simulink model "Main_bikesim"  (R2023b)
settings: Solver=FixedStepAuto  StartTime=0.0  StopTime=sim_time-0.02  FixedStep=0.005
values from neighbouring files (symbols this model uses):
  A_d = (eye(size(A))+Ts*A)    [Main_sim.m]
  Ad_t = (eye(size(A_t))+Ts*A_t)    [Main_sim.m]
  B_d = Ts*B    [Main_sim.m]
  Bd_t = B_t*Ts    [Main_sim.m]
  bike_model = 1    [Main_sim.m]
  bike_params = LoadBikeParameters(bike)    [Main_sim.m]
  C1 = [1 0 0 0 0 0 0 ... (first row only)    [Main_sim.m]
  C2 = [(-g+((-h_imu*g)/h)) 0 (-h_imu*(h*v^2-(g*lr*c)))*sin(lambda)/((lr+lf)*h^2)+(v^2)*sin(lambda)/(lr+lf) 0 ... (first row only)    [Main_sim.m]
  counter = (Ts_GPS / Ts) - 1    (= 9)    [Main_sim.m]
  D1 = [0 0 (-h_imu*lr*v)/((lr+lf)*h) 0 0 0 0]'    [Main_sim.m]
  D2 = [(-h_imu*lr*v)/((lr+lf)*h) 0 0 0 0]'    [Main_sim.m]
  e1_max = abs(-k2*e2_max/k1)    [Main_sim.m]
  g = 9.81    [Main_sim.m]
  hor_dis = 10    [Main_sim.m]
  I_balancing_outer = 0.0    (= 0)    [Main_sim.m]
  initial_state_estimate = initial_state    [Main_sim.m]
  k1 = K(1)    [Main_sim.m]
  k2 = K(2)    [Main_sim.m]
  Kalman_gain1 = Kalman_gain1'    [Main_sim.m]
  Kalman_gain2 = Kalman_gain1(4:7,3:7)    [Main_sim.m]
  P_balancing_inner = 75.5    [Main_sim.m]
  P_balancing_outer = 75.75    [Main_sim.m]
  Psiref = traj(3:end,3)    [Main_sim.m]    (also in ReferenceGenerator.m = [Psiref(1); Psiref(1); Psiref])
  ref_dis = 0.01    [Main_sim.m]
  ref_start_idx = 2    [Main_sim.m]
  T = Rz*Ry*Rx    [Main_sim.m]
  Ts = 0.01    [Main_sim.m]
  v = 1.10    (= 1.1)    [Main_sim.m]
  Xref = traj(3:end,1)    [Main_sim.m]    (also in ReferenceGenerator.m = [Xref(1); Xref])
  Yref = traj(3:end,2)    [Main_sim.m]    (also in ReferenceGenerator.m = [Yref(1); Yref])
undefined symbols (not defined in the file or in its folder): C_t, D_t, initial_state, linearized_sys, pert_deltadot_state, pert_deltadot_state_fun, pert_phidot_state, pert_phidot_state_fun, sigbuilder_block
libraries: simulink x8, slpidlib x2, eeGeneralControl x1
(part 1 of 2)
settings Model: PauseTimes=0.16  Creator=Hadi Hajieghrary  LastModifiedBy=nicholasgranlund
settings SolverCC: MaxConsecutiveMinStep=10  ZeroCrossAlgorithm=Adaptive  AlgebraicLoopSolver=TrustRegion  AutoInsertRateTranBlk=on
settings OptimizationCC: ReuseModelBlockBuffer=off
settings DebuggingCC: AlgebraicLoopMsg=none  UnconnectedInputMsg=warning  UnconnectedOutputMsg=warning  UnconnectedLineMsg=warning
settings ModelReferenceCC: EnableRefExpFcnMdlSchedulingChecks=on
settings RTWCC: GenCodeOnly=on  DLArmComputeVersion=19.05

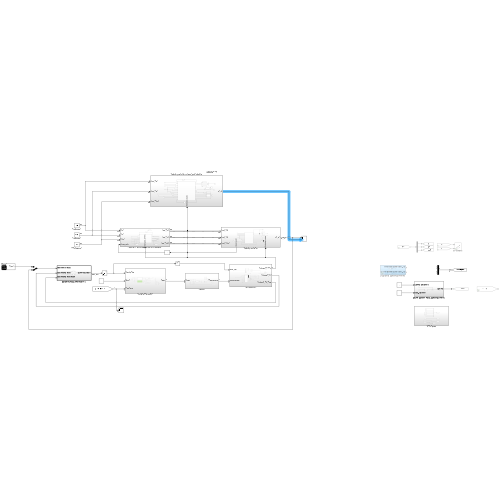
[thumbnail: Simulink's stored preview of the top-level diagram]
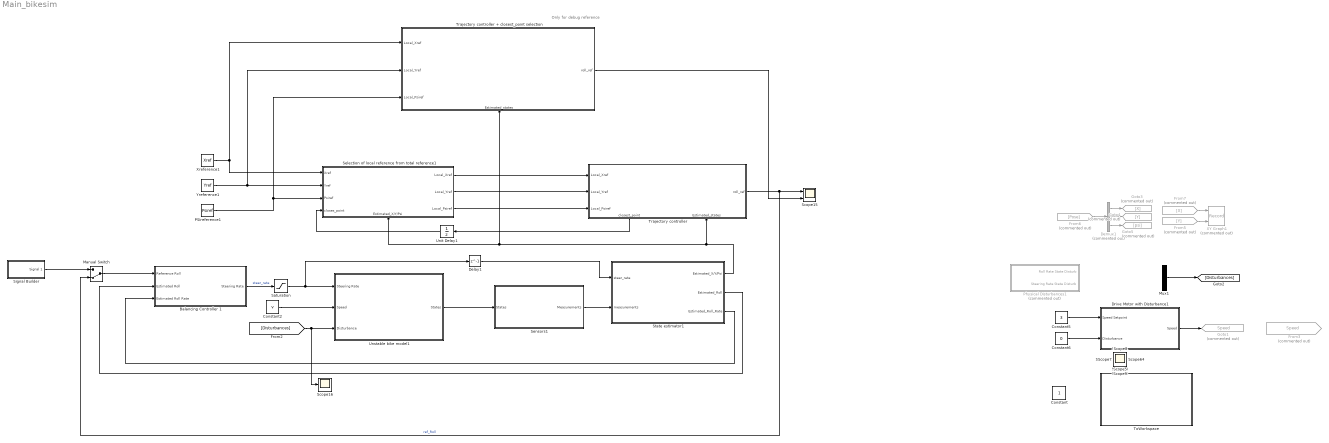
== system Main_bikesim ==
  note: Only for debug reference
  Balancing Controller 1 : Subsystem  TreatAsAtomicUnit=on  SystemSampleTime=Ts
      settings: MinAlgLoopOccurrences=on
  Constant2 : Constant  Value=v
  Constant5 : Constant  Value=3
  Constant6 : Constant  Value=0
  Delay1 : Delay  DelayLength=1  SampleTime=Ts
  Demux1 : Demux  Commented=on  Outputs=3
  Drive Motor with Disturbance1 : Subsystem
  From3 : From  Commented=on  GotoTag=Speed  TagVisibility=global
  From5 : From  Commented=on  GotoTag=Y
  From6 : From  Commented=on  GotoTag=Pose
  From7 : From  Commented=on  GotoTag=X
  Goto1 : Goto  Commented=on  GotoTag=Speed  TagVisibility=global
  Goto3 : Goto  Commented=on  GotoTag=X
  Goto4 : Goto  Commented=on  GotoTag=Y
  Goto5 : Goto  Commented=on  GotoTag=psi
  Manual Switch : ManualSwitch  CurrentSetting=0
  Mux1 : Mux  Inputs=2
  PSIreference1 : Constant  Value=Psiref
  Physical Disturbances1 : Subsystem  Commented=on
  Saturation : Saturate  UpperLimit=deg2rad(336/2)  LowerLimit=-deg2rad(336/2)
  Scope15 : Scope  NumInputPorts=2
  Scope{,1..14,16} (16 alike) : Scope
  Selection of local reference from total reference1 : Subsystem
      settings: PortSchema="{\"entries\":[{\"content\":{\"sides\":[{\"content\":{\"connectorIds\":[\"In1\",\"In2\",\"In3\",\"In4\"]},\"type\":\"ConnectorPlacement.EquallySpacedRectSide\",\"uuid\":\"b129a8ce-0ab0-4745-b919-7f1f6310ba72\"},{\"content\":{\"connectorIds\":[\"Out1\",\"Out2\",\"Out3\"],\"side\":\"RIGHT\"},\"type\":\"ConnectorPlacement.EquallySpacedRectSide\",\"uuid\":\"29e87fb1-7c56-4cac-b724-1406f2c9c629\"},{\"content\":{\"connectorIds\":[],\"side\":\"TOP\"},\"type\":\"ConnectorPlacement.EquallySpacedRectSide\",\"uuid\":\"7b58316d-0623-4272-bbb4-c0141a57ab8b\"},{\"content\":{\"connectorIds\":[\"In5\"],\"side\":\"BOTTOM\"},\"type\":\"ConnectorPlacement.EquallySpacedRectSide\",\"uuid\":\"0102ebd0-fd1a-417a-bd7a-ba724799aedf\"}]},\"type\":\"ConnectorPlacement.EquallySpacedConnector\",\"uuid\":\"fda0eb97-4558-45cb-9afe-cb94e226b238\"}],\"packageUris\":[\"http://schema.mathworks.com/mf0/Connector/R2020b\"],\"version\":\"1.0\"}"
  Sensors1 : Subsystem
  Signal Builder : Subsystem  Tag=STV Subsys  LoadFcn=sigbuilder_block('load');  StartFcn=sigbuilder_block('start');  StopFcn=sigbuilder_block('stop');  ClipboardFcn=sigbuilder_block('clipboard');  mask(Sigbuilder block){tuvar=[0:10]}
      mask help: Simulink:masks:SigbuilderBlock_MD
      mask init:
      | if ~strcmp(get_param(bdroot(gcbh),'SimulationStatus'),'stopped') tuvar = sigbuilder_block('maskInit'); end
      settings: CopyFcn=sigbuilder_block('copy');  DeleteFcn=sigbuilder_block('delete');  ModelCloseFcn=sigbuilder_block('modelClose');  PreSaveFcn=sigbuilder_block('preSave');  PauseFcn=sigbuilder_block('pause');  ContinueFcn=sigbuilder_block('continue');  NameChangeFcn=sigbuilder_block('namechange');  OpenFcn=sigbuilder_block('open',[418.8 162 550.8 400.2 ]);  CloseFcn=sigbuilder_block('close');
      mask Display: plot(0, 0, 100, 100,[2, 2, 32, 32, 2], [68, 8, 8, 68, 68],[32, 2], [38, 38], [32, 19, 2],[53, 60, 44], [32, 17, 17, 2],[16, 16, 31, 31]);txt = getActiveGroup(gcbh);text(2, 100, txt,'verticalAlignment', 'top');
  State estimator1 : Subsystem
  ToWorkspace : Subsystem
  Trajectory controller : Subsystem
      settings: PortSchema="{\"entries\":[{\"content\":{\"sides\":[{\"content\":{\"connectorIds\":[\"In1\",\"In2\",\"In3\"]},\"type\":\"ConnectorPlacement.EquallySpacedRectSide\",\"uuid\":\"e7a2fb02-f6cc-45e9-8980-79d12a8832e3\"},{\"content\":{\"connectorIds\":[\"Out1\"],\"side\":\"RIGHT\"},\"type\":\"ConnectorPlacement.EquallySpacedRectSide\",\"uuid\":\"304c1e91-f1f4-462f-993e-75a0bfc51b31\"},{\"content\":{\"connectorIds\":[],\"side\":\"TOP\"},\"type\":\"ConnectorPlacement.EquallySpacedRectSide\",\"uuid\":\"75b9e2ee-7eae-4db3-b507-7ba54d105139\"},{\"content\":{\"connectorIds\":[\"Out2\",\"In4\"],\"side\":\"BOTTOM\"},\"type\":\"ConnectorPlacement.EquallySpacedRectSide\",\"uuid\":\"8b853725-4c9a-4fb3-93ea-b9b3b3cf0d57\"}]},\"type\":\"ConnectorPlacement.EquallySpacedConnector\",\"uuid\":\"c24d7268-89b5-4c3c-b432-105407319c62\"}],\"packageUris\":[\"http://schema.mathworks.com/mf0/Connector/R2020b\"],\"version\":\"1.0\"}"
  Trajectory controller + closest_point selection : Subsystem
      settings: PortSchema="{\"entries\":[{\"content\":{\"sides\":[{\"content\":{\"connectorIds\":[\"In1\",\"In2\",\"In3\"]},\"type\":\"ConnectorPlacement.EquallySpacedRectSide\",\"uuid\":\"4e12ce37-1515-428d-8e72-ea3bf7cb0ff9\"},{\"content\":{\"connectorIds\":[\"Out1\"],\"side\":\"RIGHT\"},\"type\":\"ConnectorPlacement.EquallySpacedRectSide\",\"uuid\":\"a9718efd-1612-4f51-92cf-6f7a8bfe2bda\"},{\"content\":{\"connectorIds\":[],\"side\":\"TOP\"},\"type\":\"ConnectorPlacement.EquallySpacedRectSide\",\"uuid\":\"2b79877e-8290-4d72-b67b-1728e8961ce6\"},{\"content\":{\"connectorIds\":[\"In4\"],\"side\":\"BOTTOM\"},\"type\":\"ConnectorPlacement.EquallySpacedRectSide\",\"uuid\":\"2cd29579-a861-4f37-a88d-667717891393\"}]},\"type\":\"ConnectorPlacement.EquallySpacedConnector\",\"uuid\":\"1636a1cb-255f-43a6-9614-48f01e829aec\"}],\"packageUris\":[\"http://schema.mathworks.com/mf0/Connector/R2020b\"],\"version\":\"1.0\"}"
  Unit Delay1 : UnitDelay  InitialCondition=ref_start_idx  SampleTime=Ts  HasFrameUpgradeWarning=on
  Unstable bike model1 : Subsystem
  XY Graph1 : Record  Commented=on  FileSettingsInternal="{\"entries\":[{\"content\":{\"excelSettings\":{\"content\":{},\"type\":\"Streamout.ExcelSettings\"}},\"type\":\"Streamout.FileSettingStorage\",\"uuid\":\"\"}],\"packageUris\":[\"http:\\/\\/schema.mathworks.com\\/mf0\\/streamout_blocks\\/R2020a\"],\"version\":\"1.0\"}"  Layout=[1 1]  SignalsInternal="{\"entries\":[{\"content\":{},\"type\":\"RecordBlkView.InputSignals\",\"uuid\":\"\"}],\"packageUris\":[\"http:\\/\\/schema.mathworks.com\\/mf0\\/streamout_blocks\\/R2020a\"],\"version\":\"1.0\"}"  VisualizationBindings="{\"xyplotplugin\":{\"info\":[{\"series\":[],\"subplotID\":1}]}}"  CompatibilityTag=XY
  Xreference1 : Constant  Value=Xref
  Yreference1 : Constant  Value=Yref
  Constant : Constant  IOType=siggen
  wires:
  Yreference1/1 -> Trajectory controller + closest_point selection/2(Local_Yref), Selection of local reference from total reference1/2(Yref)
  State estimator1/1(Estimated_X/Y/Psi) -> Trajectory controller/4(Estimated_states), Selection of local reference from total reference1/5(Estimated_X/Y/Psi), Trajectory controller + closest_point selection/4(Estimated_states)
  PSIreference1/1 -> Trajectory controller + closest_point selection/3(Local_Psiref), Selection of local reference from total reference1/3(Psiref)
  Delay1/1 -> State estimator1/1(steer_rate)
  Unstable bike model1/1(States) -> Sensors1/1(States)
  Demux1/1 -> Goto3/1
  Balancing Controller 1/1(Steering Rate) -> Saturation/1  "steer_rate"
  Xreference1/1 -> Selection of local reference from total reference1/1(Xref), Trajectory controller + closest_point selection/1(Local_Xref)
  Selection of local reference from total reference1/3(Local_Psiref) -> Trajectory controller/3(Local_Psiref)
  Selection of local reference from total reference1/2(Local_Yref) -> Trajectory controller/2(Local_Yref)
  From5/1 -> XY Graph1/2
  Sensors1/1(Measurements) -> State estimator1/2(measurements)
  [Disturbances] -> Unstable bike model1/3(Disturbance), Scope16/1
  Trajectory controller/2(closest_point) -> Unit Delay1/1
  Selection of local reference from total reference1/1(Local_Xref) -> Trajectory controller/1(Local_Xref)
  State estimator1/2(Estimated_Roll) -> Balancing Controller 1/2(Estimated Roll)
  Demux1/3 -> Goto5/1
  Unit Delay1/1 -> Selection of local reference from total reference1/4(closes_point)
  Demux1/2 -> Goto4/1
  Drive Motor with Disturbance1/1(Speed) -> Goto1/1
  Mux1/1 -> [Disturbances]
  Constant5/1 -> Drive Motor with Disturbance1/1(Speed Setpoint)
  From7/1 -> XY Graph1/1
  Constant6/1 -> Drive Motor with Disturbance1/2(Disturbance)
  From6/1 -> Demux1/1
  State estimator1/3(Estimated_Roll_Rate) -> Balancing Controller 1/3(Estimated Roll Rate)
  Trajectory controller + closest_point selection/1(roll_ref) -> Scope15/2
  Manual Switch/1 -> Balancing Controller 1/1(Reference Roll)
  Signal Builder/1(Signal 1) -> Manual Switch/1
  Trajectory controller/1(roll_ref) -> Manual Switch/2, Scope15/1  "ref_Roll"
  Constant2/1 -> Unstable bike model1/2(Speed)
  Saturation/1 -> Delay1/1, Unstable bike model1/1(Steering Rate)

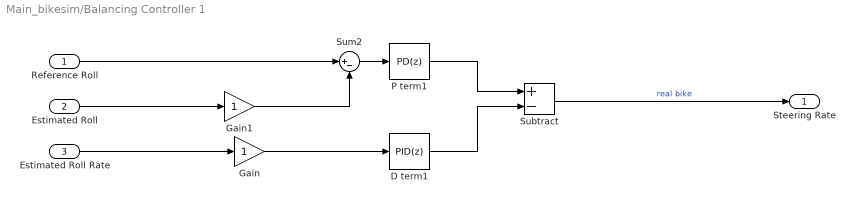
== system Main_bikesim/Balancing Controller 1 ==
  Reference Roll : Inport
  Estimated Roll : Inport  Port=2
  Estimated Roll Rate : Inport  Port=3
  D term1 : slpidlib/PID Controller  Controller=PID  Form=Parallel  TimeDomain=Discrete-time  UseExternalTs=off  SampleTime=Ts  IntegratorMethod=Forward Euler  FilterMethod=Forward Euler  ControllerParametersSource=internal  P=P_balancing_inner  I=0  UseKiTs=off  D=0  N=100  UseFilter=off  TunerSelectOption=Transfer Function Based (PID Tuner App)  InitialConditionSource=internal  InitialConditionForIntegrator=0  InitialConditionForFilter=0  DifferentiatorICPrevScaledInput=0  ExternalReset=none  TrackingMode=off  Kt=1  LimitOutput=off  SatLimitsSource=internal  UpperSaturationLimit=inf  LowerSaturationLimit=-inf  LinearizeAsGain=on  AntiWindupMode=none  Kb=1  LimitIntegrator=off  UpperIntegratorSaturationLimit=inf  LowerIntegratorSaturationLimit=-inf  POutMin=[]  POutMax=[]  IOutMin=[]  IOutMax=[]  DOutMin=[]  DOutMax=[]  NOutMin=[]  NOutMax=[]  SumOutMin=[]  SumOutMax=[]  SaturationOutMin=[]  SaturationOutMax=[]  PParamMin=[]  PParamMax=[]  IParamMin=[]  IParamMax=[]  DParamMin=[]  DParamMax=[]  NParamMin=[]  NParamMax=[]  KbParamMin=[]  KbParamMax=[]  KtParamMin=[]  KtParamMax=[]  KbOutMin=[]  KbOutMax=[]  KtOutMin=[]  KtOutMax=[]  IntegratorOutMin=[]  IntegratorOutMax=[]  FilterOutMin=[]  FilterOutMax=[]  SumI1OutMin=[]  SumI1OutMax=[]  SumI2OutMin=[]  SumI2OutMax=[]  SumI3OutMin=[]  SumI3OutMax=[]  SumI4OutMin=[]  SumI4OutMax=[]  SumDOutMin=[]  SumDOutMax=[]  DifferentiatorOutMin=[]  DifferentiatorOutMax=[]  FilterDiffOutCoefMin=[]  FilterDiffOutCoefMax=[]  ReciprocalOutMin=[]  ReciprocalOutMax=[]  SumDenOutMin=[]  SumDenOutMax=[]  SumNumOutMin=[]  SumNumOutMax=[]  DivideOutMin=[]  DivideOutMax=[]  UdiffTsProdOutMin=[]  UdiffTsProdOutMax=[]  NTsProdOutMin=[]  NTsProdOutMax=[]  UintegralTsProdOutMin=[]  UintegralTsProdOutMax=[]  UngainTsProdOutMin=[]  UngainTsProdOutMax=[]  ClampingZeroOutDataTypeStr=Inherit: Inherit via back propagation  ClampingZeroOutMin=[]  ClampingZeroOutMax=[]  FilterDenConstantOutDataTypeStr=Inherit: Inherit via back propagation  FilterDenConstantOutMin=[]  FilterDenConstantOutMax=[]  PCopyOutDataTypeStr=Inherit: Inherit via back propagation  PCopyOutMin=[]  PCopyOutMax=[]  NCopyOutDataTypeStr=Inherit: Inherit via back propagation  NCopyOutMin=[]  NCopyOutMax=[]  IntegratorContinuousStateAttributes=''  IntegratorStateMustResolveToSignalObject=off  IntegratorRTWStateStorageClass=Auto  FilterContinuousStateAttributes=''  FilterStateMustResolveToSignalObject=off  FilterRTWStateStorageClass=Auto  ParallelPVariant=InternalParameters  IdealPVariant=Disabled  IVariant=InternalParameters  DVariant=InternalParameters  IntegratorVariant=Discrete  SatVariant=Disabled  AWVariant=Passthrough  PCopyVariant=Disabled  TRVariant=Disabled  FdbkBlocksVariant=Forward  IdealPFdbkVariant=Disabled  SatFdbkVariant=Disabled  DerivativeFilterVariant=Differentiator  NVariant=Passthrough  NCopyVariant=Disabled_SignalSpec  FilterICVariant=InternalICsDifferentiator  IntegratorICVariant=InternalICs  ExternalResetVariant=Disabled  TRSumVariant=Passthrough  SumFdbkVariant=Disabled  SumVariant=Sum_PID  TsampFilterVariant=InternalTs  TsampNgainVariant=Passthrough  TsampIntegralVariant=Disabled_SignalSpec  ExternalSaturationOutDataTypeStr=Inherit: Same as second input
  Gain : Gain
  Gain1 : Gain
  P term1 : slpidlib/PID Controller  Controller=PD  Form=Parallel  TimeDomain=Discrete-time  UseExternalTs=off  SampleTime=Ts  IntegratorMethod=Forward Euler  FilterMethod=Forward Euler  ControllerParametersSource=internal  P=P_balancing_outer  I=I_balancing_outer  UseKiTs=off  D=0  N=100  UseFilter=off  TunerSelectOption=Transfer Function Based (PID Tuner App)  InitialConditionSource=internal  InitialConditionForIntegrator=0  InitialConditionForFilter=0  DifferentiatorICPrevScaledInput=0  ExternalReset=none  TrackingMode=off  Kt=1  LimitOutput=off  SatLimitsSource=internal  UpperSaturationLimit=inf  LowerSaturationLimit=-inf  LinearizeAsGain=on  AntiWindupMode=none  Kb=1  LimitIntegrator=off  UpperIntegratorSaturationLimit=inf  LowerIntegratorSaturationLimit=-inf  POutMin=[]  POutMax=[]  IOutMin=[]  IOutMax=[]  DOutMin=[]  DOutMax=[]  NOutMin=[]  NOutMax=[]  SumOutMin=[]  SumOutMax=[]  SaturationOutMin=[]  SaturationOutMax=[]  PParamMin=[]  PParamMax=[]  IParamMin=[]  IParamMax=[]  DParamMin=[]  DParamMax=[]  NParamMin=[]  NParamMax=[]  KbParamMin=[]  KbParamMax=[]  KtParamMin=[]  KtParamMax=[]  KbOutMin=[]  KbOutMax=[]  KtOutMin=[]  KtOutMax=[]  IntegratorOutMin=[]  IntegratorOutMax=[]  FilterOutMin=[]  FilterOutMax=[]  SumI1OutMin=[]  SumI1OutMax=[]  SumI2OutMin=[]  SumI2OutMax=[]  SumI3OutMin=[]  SumI3OutMax=[]  SumI4OutMin=[]  SumI4OutMax=[]  SumDOutMin=[]  SumDOutMax=[]  DifferentiatorOutMin=[]  DifferentiatorOutMax=[]  FilterDiffOutCoefMin=[]  FilterDiffOutCoefMax=[]  ReciprocalOutMin=[]  ReciprocalOutMax=[]  SumDenOutMin=[]  SumDenOutMax=[]  SumNumOutMin=[]  SumNumOutMax=[]  DivideOutMin=[]  DivideOutMax=[]  UdiffTsProdOutMin=[]  UdiffTsProdOutMax=[]  NTsProdOutMin=[]  NTsProdOutMax=[]  UintegralTsProdOutMin=[]  UintegralTsProdOutMax=[]  UngainTsProdOutMin=[]  UngainTsProdOutMax=[]  ClampingZeroOutDataTypeStr=Inherit: Inherit via back propagation  ClampingZeroOutMin=[]  ClampingZeroOutMax=[]  FilterDenConstantOutDataTypeStr=Inherit: Inherit via back propagation  FilterDenConstantOutMin=[]  FilterDenConstantOutMax=[]  PCopyOutDataTypeStr=Inherit: Inherit via back propagation  PCopyOutMin=[]  PCopyOutMax=[]  NCopyOutDataTypeStr=Inherit: Inherit via back propagation  NCopyOutMin=[]  NCopyOutMax=[]  IntegratorContinuousStateAttributes=''  IntegratorStateMustResolveToSignalObject=off  IntegratorRTWStateStorageClass=Auto  FilterContinuousStateAttributes=''  FilterStateMustResolveToSignalObject=off  FilterRTWStateStorageClass=Auto  ParallelPVariant=InternalParameters  IdealPVariant=Disabled  IVariant=Disabled  DVariant=InternalParameters  IntegratorVariant=Disabled  SatVariant=Disabled  AWVariant=Disabled  PCopyVariant=Disabled  TRVariant=Disabled  FdbkBlocksVariant=Forward  IdealPFdbkVariant=Disabled  SatFdbkVariant=Disabled  DerivativeFilterVariant=Differentiator  NVariant=Passthrough  NCopyVariant=Disabled_SignalSpec  FilterICVariant=InternalICsDifferentiator  IntegratorICVariant=Disabled  ExternalResetVariant=Disabled  TRSumVariant=Passthrough  SumFdbkVariant=Disabled  SumVariant=Sum_PD  TsampFilterVariant=InternalTs  TsampNgainVariant=Passthrough  TsampIntegralVariant=Disabled_SignalSpec  ExternalSaturationOutDataTypeStr=Inherit: Same as second input
  Subtract : Sum  Inputs=+-
  Sum2 : Sum  Inputs=|+-
  Steering Rate : Outport
  wires:
  Sum2/1 -> P term1/1
  D term1/1 -> Subtract/2
  P term1/1 -> Subtract/1
  Estimated Roll Rate/1 -> Gain/1
  Subtract/1 -> Steering Rate/1  "real bike"
  Estimated Roll/1 -> Gain1/1
  Reference Roll/1 -> Sum2/1
  Gain/1 -> D term1/1
  Gain1/1 -> Sum2/2

== system Main_bikesim/Drive Motor with Disturbance1 ==
  Speed Setpoint : Inport
  Disturbance : Inport  Port=2
  Sum2 : Sum  Inputs=++|
  Transfer Fcn : TransferFcn  Denominator=[2 1]
  Speed : Outport
  wires:
  Sum2/1 -> Speed/1
  Transfer Fcn/1 -> Sum2/2
  Speed Setpoint/1 -> Transfer Fcn/1
  Disturbance/1 -> Sum2/1

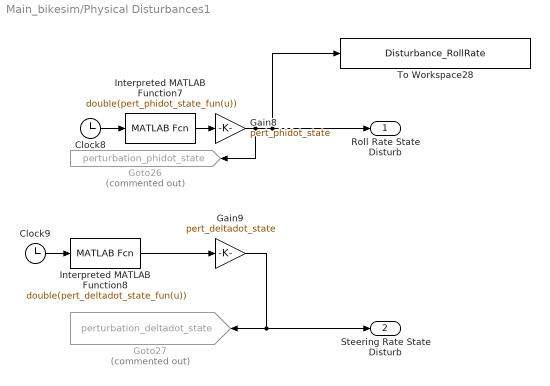
== system Main_bikesim/Physical Disturbances1 ==
  Clock8 : Clock
  Clock9 : Clock
  Gain8 : Gain  Gain=pert_phidot_state
  Gain9 : Gain  Gain=pert_deltadot_state
  Goto26 : Goto  Commented=on  GotoTag=perturbation_phidot_state  TagVisibility=global
  Goto27 : Goto  Commented=on  GotoTag=perturbation_deltadot_state  TagVisibility=global
  Interpreted MATLAB Function7 : MATLABFcn  MATLABFcn=double(pert_phidot_state_fun(u))
  Interpreted MATLAB Function8 : MATLABFcn  MATLABFcn=double(pert_deltadot_state_fun(u))
  To Workspace28 : ToWorkspace  VariableName=Disturbance_RollRate  SaveFormat=Timeseries  SampleTime=-1
  Roll Rate State Disturb : Outport
  Steering Rate State Disturb : Outport  Port=2
  wires:
  Interpreted MATLAB Function7/1 -> Gain8/1
  Clock8/1 -> Interpreted MATLAB Function7/1
  Gain8/1 -> Goto26/1, Roll Rate State Disturb/1, To Workspace28/1
  Interpreted MATLAB Function8/1 -> Gain9/1
  Clock9/1 -> Interpreted MATLAB Function8/1
  Gain9/1 -> Steering Rate State Disturb/1, Goto27/1

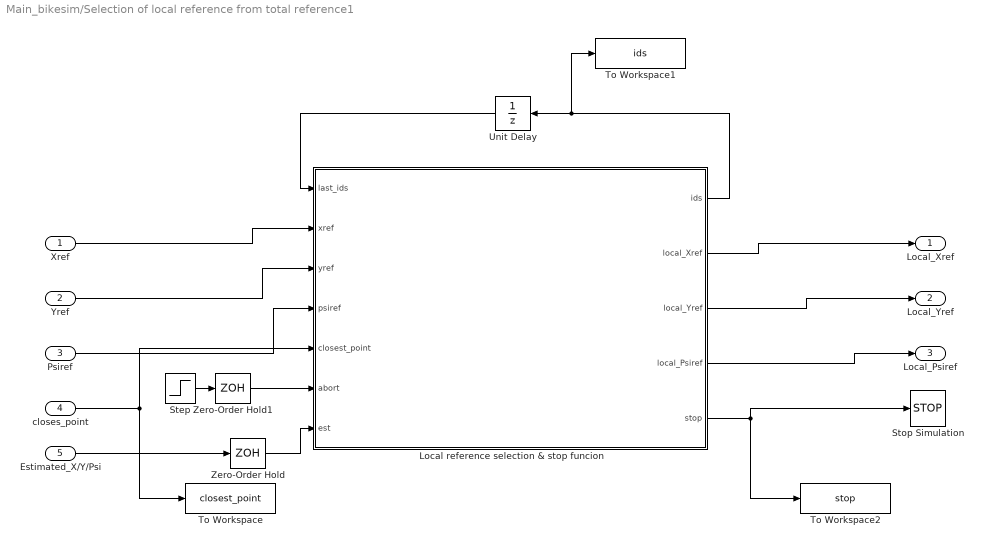
== system Main_bikesim/Selection of local reference from total reference1 ==
  Xref : Inport
  Yref : Inport  Port=2
  Psiref : Inport  Port=3
  closes_point : Inport  Port=4
  Estimated_X/Y/Psi : Inport  Port=5
  Local reference selection & stop funcion : MATLAB Function  TreatAsAtomicUnit=on
  Step : Step  Time=20  After=0  SampleTime=0
  Stop Simulation : Stop
  To Workspace : ToWorkspace  VariableName=closest_point  SaveFormat=Timeseries  SampleTime=-1
  To Workspace1 : ToWorkspace  VariableName=ids  SaveFormat=Timeseries  SampleTime=-1
  To Workspace2 : ToWorkspace  VariableName=stop  SaveFormat=Timeseries  SampleTime=-1
  Unit Delay : UnitDelay  InitialCondition=1  SampleTime=Ts  HasFrameUpgradeWarning=on
  Zero-Order Hold : ZeroOrderHold  SampleTime=-1
  Zero-Order Hold1 : ZeroOrderHold  SampleTime=-1
  Local_Xref : Outport
  Local_Yref : Outport  Port=2
  Local_Psiref : Outport  Port=3
  wires:
  Local reference selection & stop funcion/1(ids) -> To Workspace1/1, Unit Delay/1
  Unit Delay/1 -> Local reference selection & stop funcion/1(last_ids)
  closes_point/1 -> To Workspace/1, Local reference selection & stop funcion/5(closest_point)
  Xref/1 -> Local reference selection & stop funcion/2(xref)
  Yref/1 -> Local reference selection & stop funcion/3(yref)
  Psiref/1 -> Local reference selection & stop funcion/4(psiref)
  Local reference selection & stop funcion/5(stop) -> Stop Simulation/1, To Workspace2/1
  Local reference selection & stop funcion/2(local_Xref) -> Local_Xref/1
  Local reference selection & stop funcion/3(local_Yref) -> Local_Yref/1
  Local reference selection & stop funcion/4(local_Psiref) -> Local_Psiref/1
  Estimated_X/Y/Psi/1 -> Zero-Order Hold/1
  Zero-Order Hold/1 -> Local reference selection & stop funcion/7(est)
  Zero-Order Hold1/1 -> Local reference selection & stop funcion/6(abort)
  Step/1 -> Zero-Order Hold1/1

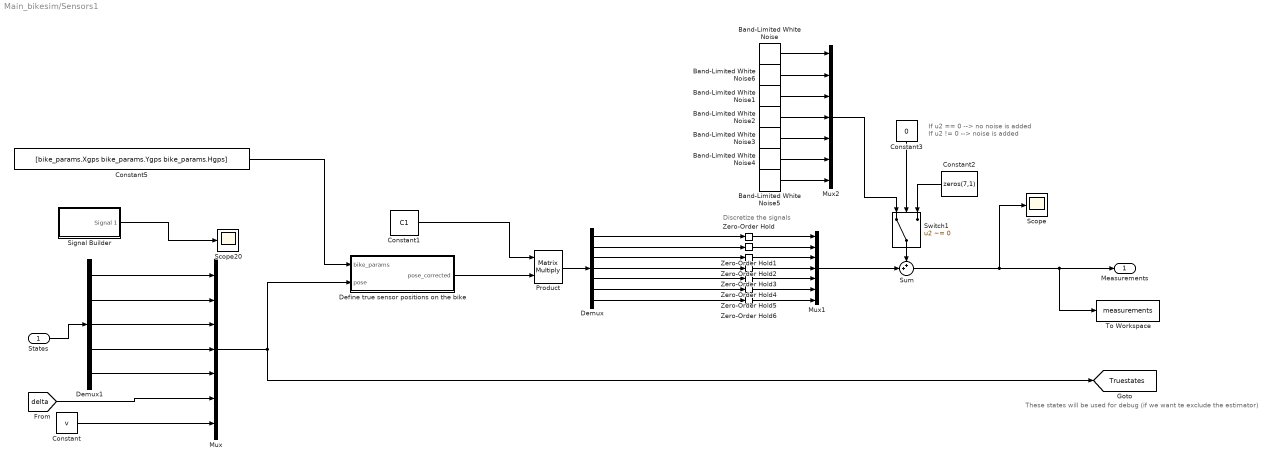
== system Main_bikesim/Sensors1 ==
  note: These states will be used for debug (if we want te exclude the estimator)
  note: Discretize the signals
  note: If u2 == 0 --> no noise is added
      | If u2 != 0 --> noise is added
  States : Inport
  Band-Limited White Noise : simulink/Sources/Band-Limited White Noise  Cov=0.001  Ts=Ts  seed=[23341]
  Band-Limited White Noise{1..6} (6 alike) : simulink/Sources/Band-Limited White Noise  Cov=0  Ts=Ts  seed=[23341]
  Constant : Constant  Value=v
  Constant1 : Constant  Value=C1
  Constant2 : Constant  Value=zeros(7,1)
  Constant3 : Constant  Value=0
  Constant5 : Constant  Value=[bike_params.Xgps bike_params.Ygps bike_params.Hgps]
  Define true sensor positions on the bike : MATLAB Function  TreatAsAtomicUnit=on
  Demux : Demux  Outputs=7
  Demux1 : Demux  Outputs=5
  Mux : Mux  Inputs=7
  Mux1 : Mux  Inputs=7
  Mux2 : Mux  Inputs=7
  Product : Product  Multiplication=Matrix(*)
  Scope : Scope
  Scope20 : Scope
  Signal Builder : Subsystem  Tag=STV Subsys  LoadFcn=sigbuilder_block('load');  StartFcn=sigbuilder_block('start');  StopFcn=sigbuilder_block('stop');  ClipboardFcn=sigbuilder_block('clipboard');  mask(Sigbuilder block){tuvar=[0:10]}
      mask help: Simulink:masks:SigbuilderBlock_MD
      mask init:
      | if ~strcmp(get_param(bdroot(gcbh),'SimulationStatus'),'stopped') tuvar = sigbuilder_block('maskInit'); end
      settings: CopyFcn=sigbuilder_block('copy');  DeleteFcn=sigbuilder_block('delete');  ModelCloseFcn=sigbuilder_block('modelClose');  PreSaveFcn=sigbuilder_block('preSave');  PauseFcn=sigbuilder_block('pause');  ContinueFcn=sigbuilder_block('continue');  NameChangeFcn=sigbuilder_block('namechange');  OpenFcn=sigbuilder_block('open',[5.4 36 1141.2 516.6 ]);  CloseFcn=sigbuilder_block('close');
      mask Display: plot(0, 0, 100, 100,[2, 2, 32, 32, 2], [68, 8, 8, 68, 68],[32, 2], [38, 38], [32, 19, 2],[53, 60, 44], [32, 17, 17, 2],[16, 16, 31, 31]);txt = getActiveGroup(gcbh);text(2, 100, txt,'verticalAlignment', 'top');
  Sum : Sum  Inputs=++|
  Switch1 : Switch  Criteria=u2 ~= 0  SaturateOnIntegerOverflow=off  InputSameDT=off
  To Workspace : ToWorkspace  VariableName=measurements  SaveFormat=Timeseries  SampleTime=-1
  Zero-Order Hold : ZeroOrderHold  SampleTime=10*Ts
  Zero-Order Hold1 : ZeroOrderHold  SampleTime=10*Ts
  Zero-Order Hold{2..6} (5 alike) : ZeroOrderHold  SampleTime=Ts
  Measurements : Outport
  tag scope: Truestates=global
  wires:
  Mux/1 -> Define true sensor positions on the bike/2(pose), [Truestates]
  Constant1/1 -> Product/1
  Switch1/1 -> Sum/1
  Constant2/1 -> Switch1/3
  Constant3/1 -> Switch1/2
  Mux1/1 -> Sum/2
  Product/1 -> Demux/1
  Demux/2 -> Zero-Order Hold1/1
  Demux/4 -> Zero-Order Hold3/1
  Demux/5 -> Zero-Order Hold4/1
  Demux/6 -> Zero-Order Hold5/1
  Demux/7 -> Zero-Order Hold6/1
  Zero-Order Hold/1 -> Mux1/1
  Zero-Order Hold1/1 -> Mux1/2
  Zero-Order Hold2/1 -> Mux1/3
  Zero-Order Hold3/1 -> Mux1/4
  Zero-Order Hold4/1 -> Mux1/5
  Zero-Order Hold5/1 -> Mux1/6
  Zero-Order Hold6/1 -> Mux1/7
  Sum/1 -> Scope/1, To Workspace/1, Measurements/1
  Demux/1 -> Zero-Order Hold/1
  Define true sensor positions on the bike/1(pose_corrected) -> Product/2
  Constant5/1 -> Define true sensor positions on the bike/1(bike_params)
  States/1 -> Demux1/1
  Constant/1 -> Mux/7
  Demux1/1 -> Mux/1
  Demux1/2 -> Mux/2
  Demux1/5 -> Mux/5
  Demux1/4 -> Mux/4
  Demux1/3 -> Mux/3
  [delta] -> Mux/6
  Mux2/1 -> Switch1/1
  Band-Limited White Noise/1 -> Mux2/1
  Band-Limited White Noise5/1 -> Mux2/7
  Band-Limited White Noise4/1 -> Mux2/6
  Band-Limited White Noise3/1 -> Mux2/5
  Band-Limited White Noise2/1 -> Mux2/4
  Band-Limited White Noise1/1 -> Mux2/3
  Band-Limited White Noise6/1 -> Mux2/2
  Signal Builder/1(Signal 1) -> Scope20/1
  Demux/3 -> Zero-Order Hold2/1

== system Main_bikesim/Signal Builder ==
  Demux : Demux  Tag=STV Demux  Outputs=1
      settings: DisplayOption=none
  FromWs : FromWorkspace  Tag=STV FromWs  VariableName=tuvar
      SigBuilderData=|
      | common.afterFinalStr = 'Extrapolate'
      | common.sampleTime = 0
      | dataSet.timeRange = [0 10]
      | dataSet.name = 'Group 1'
      | sbobj.Groups.Name = 'Group 1'
      | sbobj.Groups.Signals.Name = 'Signal 1'
      | sbobj.Groups.Signals.XData = [0 4 6 10]
      | sbobj.Groups.Signals.YData = [0 0 0 0]
  Signal 1 : Outport  Tag=STV Outport
  wires:
  Demux/1 -> Signal 1/1
  FromWs/1 -> Demux/1

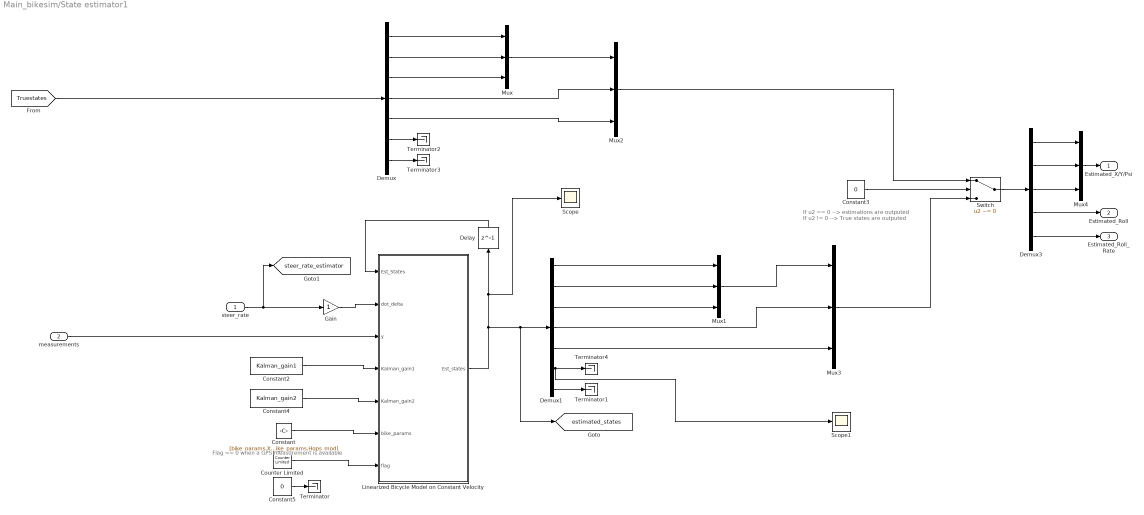
== system Main_bikesim/State estimator1 ==
  note: Flag == 0 when a GPS measurement is available
  note: If u2 == 0 --> estimations are outputed
      | If u2 != 0 --> True states are outputed
  steer_rate : Inport
  measurements : Inport  Port=2
  Constant : Constant  Value=[bike_params.Xgps_mod bike_params.Ygps_mod bike_params.Hgps_mod]
  Constant2 : Constant  Value=Kalman_gain1  SampleTime=Ts
  Constant3 : Constant  Value=0
  Constant4 : Constant  Value=Kalman_gain2  SampleTime=Ts
  Constant5 : Constant  Value=0
  Counter Limited : simulink/Sources/Counter Limited  uplimit=counter  tsamp=Ts
  Delay : Delay  DelayLength=1  InitialCondition=[initial_state_estimate.x initial_state_estimate.y initial_state_estimate.heading initial_state.roll initial_state.roll_rate initial_state.steering v]  SampleTime=Ts
  Demux : Demux  Outputs=7
  Demux1 : Demux  Outputs=7
  Demux3 : Demux  Outputs=5
  Gain : Gain
  Linearized Bicycle Model on Constant Velocity : MATLAB Function  TreatAsAtomicUnit=on
  Mux{,1..4} (5 alike) : Mux  Inputs=3
  Scope : Scope
  Scope1 : Scope
  Switch : Switch  Criteria=u2 ~= 0  SaturateOnIntegerOverflow=off  InputSameDT=off
  Terminator{,1..4} (5 alike) : Terminator
  Estimated_X/Y/Psi : Outport  VectorParamsAs1DForOutWhenUnconnected=off
  Estimated_Roll : Outport  Port=2  VectorParamsAs1DForOutWhenUnconnected=off
  Estimated_Roll_Rate : Outport  Port=3  VectorParamsAs1DForOutWhenUnconnected=off
  tag scope: estimated_states=global, steer_rate_estimator=global
  wires:
  Demux/3 -> Mux/3
  Gain/1 -> Linearized Bicycle Model on Constant Velocity/2(dot_delta)
  Demux1/5 -> Mux3/3
  Delay/1 -> Linearized Bicycle Model on Constant Velocity/1(Est_States)
  steer_rate/1 -> [steer_rate_estimator], Gain/1
  Demux1/2 -> Mux1/2
  Demux/1 -> Mux/1
  Demux1/1 -> Mux1/1
  Demux/2 -> Mux/2
  Demux1/7 -> Terminator1/1
  Demux/7 -> Terminator3/1
  Demux/6 -> Terminator2/1
  Mux/1 -> Mux2/1
  Mux2/1 -> Switch/1
  Mux3/1 -> Switch/3
  Constant3/1 -> Switch/2
  Demux/4 -> Mux2/2
  Demux/5 -> Mux2/3
  Mux1/1 -> Mux3/1
  Demux1/4 -> Mux3/2
  Switch/1 -> Demux3/1
  Demux3/1 -> Mux4/1
  Demux3/2 -> Mux4/2
  Demux3/3 -> Mux4/3
  Mux4/1 -> Estimated_X/Y/Psi/1
  Demux3/4 -> Estimated_Roll/1
  Demux3/5 -> Estimated_Roll_Rate/1
  Constant2/1 -> Linearized Bicycle Model on Constant Velocity/4(Kalman_gain1)
  Constant4/1 -> Linearized Bicycle Model on Constant Velocity/5(Kalman_gain2)
  Counter Limited/1 -> Linearized Bicycle Model on Constant Velocity/7(flag)
  Demux1/3 -> Mux1/3
  Constant5/1 -> Terminator/1
  Constant/1 -> Linearized Bicycle Model on Constant Velocity/6(bike_params)
  measurements/1 -> Linearized Bicycle Model on Constant Velocity/3(y)
  [Truestates] -> Demux/1
  Linearized Bicycle Model on Constant Velocity/1(Est_states) -> Scope/1, Delay/1, [estimated_states], Demux1/1
  Demux1/6 -> Scope1/1, Terminator4/1

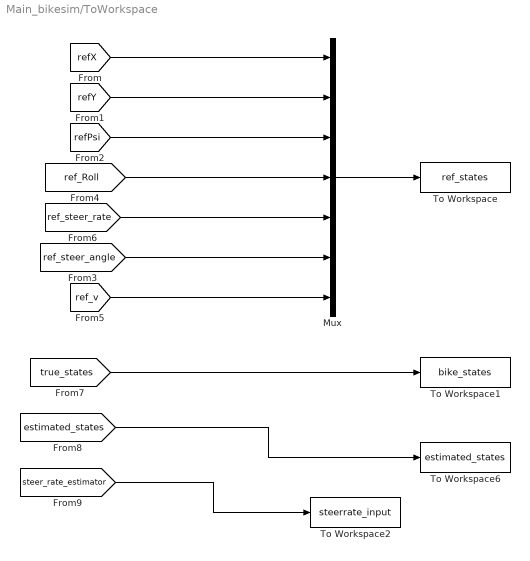
== system Main_bikesim/ToWorkspace ==
  Mux : Mux  Inputs=7
  To Workspace : ToWorkspace  VariableName=ref_states  SaveFormat=Timeseries  SampleTime=-1
  To Workspace1 : ToWorkspace  VariableName=bike_states  SaveFormat=Timeseries  SampleTime=-1
  To Workspace2 : ToWorkspace  VariableName=steerrate_input  SaveFormat=Timeseries  SampleTime=-1
  To Workspace6 : ToWorkspace  VariableName=estimated_states  SaveFormat=Timeseries  SampleTime=-1
  wires:
  [refX] -> Mux/1
  [refY] -> Mux/2
  [refPsi] -> Mux/3
  [ref_Roll] -> Mux/4
  Mux/1 -> To Workspace/1
  [true_states] -> To Workspace1/1
  [ref_v] -> Mux/7
  [ref_steer_angle] -> Mux/6
  [ref_steer_rate] -> Mux/5
  [estimated_states] -> To Workspace6/1
  [steer_rate_estimator] -> To Workspace2/1

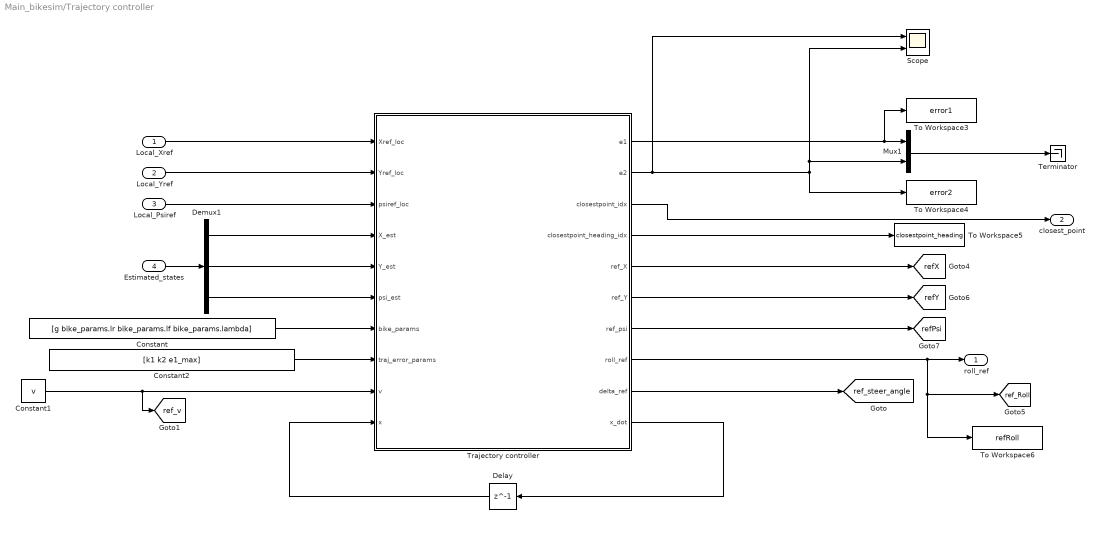
== system Main_bikesim/Trajectory controller ==
  Local_Xref : Inport
  Local_Yref : Inport  Port=2
  Local_Psiref : Inport  Port=3
  Estimated_states : Inport  Port=4
  Constant : Constant  Value=[g bike_params.lr bike_params.lf bike_params.lambda]
  Constant1 : Constant  Value=v
  Constant2 : Constant  Value=[k1 k2 e1_max]
  Delay : Delay  DelayLength=1  SampleTime=Ts
  Demux1 : Demux  Outputs=3
  Mux1 : Mux  Inputs=2
  Scope : Scope  NumInputPorts=2
  Terminator : Terminator
  To Workspace3 : ToWorkspace  VariableName=error1  SaveFormat=Timeseries  SampleTime=-1
  To Workspace4 : ToWorkspace  VariableName=error2  SaveFormat=Timeseries  SampleTime=-1
  To Workspace5 : ToWorkspace  VariableName=closestpoint_heading  SaveFormat=Timeseries  SampleTime=-1
  To Workspace6 : ToWorkspace  VariableName=refRoll  SaveFormat=Timeseries  SampleTime=-1
  Trajectory controller : MATLAB Function  TreatAsAtomicUnit=on
  roll_ref : Outport
  closest_point : Outport  Port=2
  tag scope: refPsi=global, refX=global, refY=global, ref_Roll=global, ref_steer_angle=global, ref_v=global
  wires:
  Demux1/3 -> Trajectory controller/6(psi_est)
  Trajectory controller/3(closestpoint_idx) -> closest_point/1
  Trajectory controller/4(closestpoint_heading_idx) -> To Workspace5/1
  Estimated_states/1 -> Demux1/1
  Trajectory controller/2(e2) -> Mux1/2, Scope/2, To Workspace4/1, Scope/1
  Local_Xref/1 -> Trajectory controller/1(Xref_loc)
  Local_Psiref/1 -> Trajectory controller/3(psiref_loc)
  Mux1/1 -> Terminator/1
  Trajectory controller/6(ref_Y) -> [refY]
  Demux1/2 -> Trajectory controller/5(Y_est)
  Local_Yref/1 -> Trajectory controller/2(Yref_loc)
  Demux1/1 -> Trajectory controller/4(X_est)
  Trajectory controller/5(ref_X) -> [refX]
  Trajectory controller/7(ref_psi) -> [refPsi]
  Trajectory controller/1(e1) -> To Workspace3/1, Mux1/1
  Constant1/1 -> [ref_v], Trajectory controller/9(v)
  Constant/1 -> Trajectory controller/7(bike_params)
  Constant2/1 -> Trajectory controller/8(traj_error_params)
  Trajectory controller/8(roll_ref) -> roll_ref/1, To Workspace6/1, [ref_Roll]
  Trajectory controller/10(x_dot) -> Delay/1
  Delay/1 -> Trajectory controller/10(x)
  Trajectory controller/9(delta_ref) -> [ref_steer_angle]

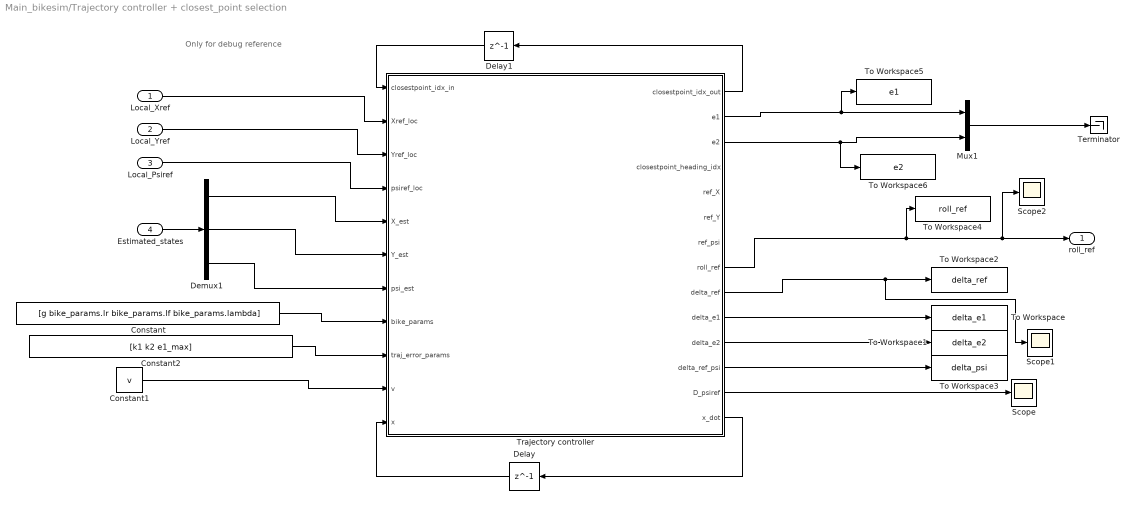
== system Main_bikesim/Trajectory controller + closest_point selection ==
  note: Only for debug reference
  Local_Xref : Inport
  Local_Yref : Inport  Port=2
  Local_Psiref : Inport  Port=3
  Estimated_states : Inport  Port=4
  Constant : Constant  Value=[g bike_params.lr bike_params.lf bike_params.lambda]
  Constant1 : Constant  Value=v
  Constant2 : Constant  Value=[k1 k2 e1_max]
  Delay : Delay  DelayLength=1  SampleTime=Ts
  Delay1 : Delay  DelayLength=1  InitialCondition=2  SampleTime=Ts
  Demux1 : Demux  Outputs=3
  Mux1 : Mux  Inputs=2
  Scope : Scope
  Scope1 : Scope
  Scope2 : Scope
  Terminator : Terminator
  To Workspace : ToWorkspace  VariableName=delta_e1  SaveFormat=Timeseries  SampleTime=-1
  To Workspace1 : ToWorkspace  VariableName=delta_e2  SaveFormat=Timeseries  SampleTime=-1
  To Workspace2 : ToWorkspace  VariableName=delta_ref  SaveFormat=Timeseries  SampleTime=-1
  To Workspace3 : ToWorkspace  VariableName=delta_psi  SaveFormat=Timeseries  SampleTime=-1
  To Workspace4 : ToWorkspace  VariableName=roll_ref  SaveFormat=Timeseries  SampleTime=-1
  To Workspace5 : ToWorkspace  VariableName=e1  SaveFormat=Timeseries  SampleTime=-1
  To Workspace6 : ToWorkspace  VariableName=e2  SaveFormat=Timeseries  SampleTime=-1
  Trajectory controller : MATLAB Function  TreatAsAtomicUnit=on
  roll_ref : Outport
  wires:
  Mux1/1 -> Terminator/1
  Trajectory controller/14(x_dot) -> Delay/1
  Trajectory controller/8(roll_ref) -> To Workspace4/1, Scope2/1, roll_ref/1
  Constant2/1 -> Trajectory controller/9(traj_error_params)
  Constant/1 -> Trajectory controller/8(bike_params)
  Estimated_states/1 -> Demux1/1
  Trajectory controller/2(e1) -> To Workspace5/1, Mux1/1
  Constant1/1 -> Trajectory controller/10(v)
  Local_Yref/1 -> Trajectory controller/3(Yref_loc)
  Local_Psiref/1 -> Trajectory controller/4(psiref_loc)
  Demux1/1 -> Trajectory controller/5(X_est)
  Demux1/2 -> Trajectory controller/6(Y_est)
  Delay/1 -> Trajectory controller/11(x)
  Local_Xref/1 -> Trajectory controller/2(Xref_loc)
  Trajectory controller/3(e2) -> To Workspace6/1, Mux1/2
  Demux1/3 -> Trajectory controller/7(psi_est)
  Trajectory controller/1(closestpoint_idx_out) -> Delay1/1
  Delay1/1 -> Trajectory controller/1(closestpoint_idx_in)
  Trajectory controller/10(delta_e1) -> To Workspace/1
  Trajectory controller/11(delta_e2) -> To Workspace1/1
  Trajectory controller/12(delta_ref_psi) -> To Workspace3/1
  Trajectory controller/13(D_psiref) -> Scope/1
  Trajectory controller/9(delta_ref) -> Scope1/1, To Workspace2/1

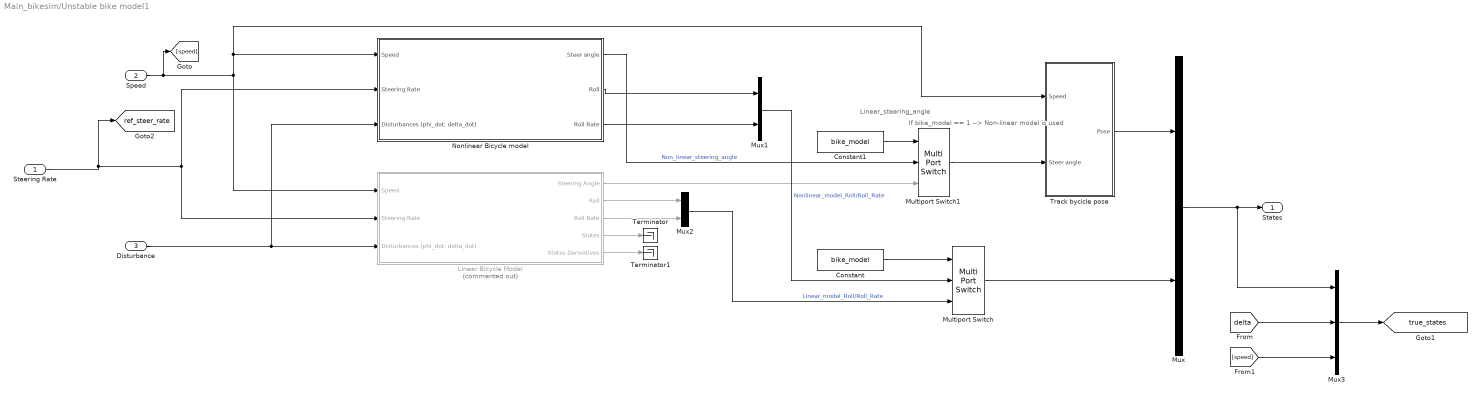
== system Main_bikesim/Unstable bike model1 ==
  note: If bike_model == 1 --> Non-linear model is used
  note: Linear_steering_angle
  Steering Rate : Inport
  Speed : Inport  Port=2
  Disturbance : Inport  Port=3
  Constant : Constant  Value=bike_model
  Constant1 : Constant  Value=bike_model
  Linear Bicycle Model : Subsystem  Commented=on  mask{Parameters=bike_params, linearized_sys=linearized_sys, Initial_State=initial_state}
      mask prompts: linearized_sys "Linearized System"; Initial_State "Initial State"
  Multiport Switch : MultiPortSwitch  Inputs=2  SaturateOnIntegerOverflow=off  InputSameDT=off
  Multiport Switch1 : MultiPortSwitch  Inputs=2  SaturateOnIntegerOverflow=off  InputSameDT=off
  Mux : Mux  Inputs=2
  Mux1 : Mux  Inputs=2
  Mux2 : Mux  Inputs=2
  Mux3 : Mux  Inputs=3
  Nonlinear Bicycle model : Subsystem
  Terminator : Terminator
  Terminator1 : Terminator
  Track bycicle pose : Subsystem
  States : Outport
  tag scope: ref_steer_rate=global, true_states=global
  wires:
  Steering Rate/1 -> Nonlinear Bicycle model/2(Steering Rate), Linear Bicycle Model/2(Steering Rate), [ref_steer_rate]
  Constant/1 -> Multiport Switch/1
  Nonlinear Bicycle model/3(Roll Rate) -> Mux1/2
  Nonlinear Bicycle model/1(Steer angle) -> Multiport Switch1/2  "Non_linear_steering_angle"
  Linear Bicycle Model/2(Roll) -> Mux2/1
  Linear Bicycle Model/3(Roll Rate) -> Mux2/2
  Linear Bicycle Model/1(Steering Angle) -> Multiport Switch1/3
  Mux1/1 -> Multiport Switch/2  "Nonlinear_model_Roll/Roll_Rate"
  Mux2/1 -> Multiport Switch/3  "Linear_model_Roll/Roll_Rate"
  Constant1/1 -> Multiport Switch1/1
  Mux/1 -> Mux3/1, States/1
  Multiport Switch/1 -> Mux/2
  Speed/1 -> [speed], Track bycicle pose/1(Speed), Nonlinear Bicycle model/1(Speed), Linear Bicycle Model/1(Speed)
  Disturbance/1 -> Nonlinear Bicycle model/3(Disturbances (phi_dot; delta_dot)), Linear Bicycle Model/3(Disturbances (phi_dot; delta_dot))
  Linear Bicycle Model/4(States) -> Terminator/1
  Linear Bicycle Model/5(States Derivatives) -> Terminator1/1
  Track bycicle pose/1(Pose) -> Mux/1
  [delta] -> Mux3/2
  [speed] -> Mux3/3
  Mux3/1 -> [true_states]
  Nonlinear Bicycle model/2(Roll) -> Mux1/1
  Multiport Switch1/1 -> Track bycicle pose/2(Steer angle)

== system Main_bikesim/Sensors1/Signal Builder ==
  Demux : Demux  Tag=STV Demux  Outputs=1
      settings: DisplayOption=none
  FromWs : FromWorkspace  Tag=STV FromWs  VariableName=tuvar
      SigBuilderData=|
      | common.afterFinalStr = 'Extrapolate'
      | common.sampleTime = '0'
      | dataSet.timeRange = [0 100]
      | dataSet.name = 'Group 1'
      | sbobj.Groups.Name = 'Group 1'
      | sbobj.Groups.Signals.Name = 'Signal 1'
      | sbobj.Groups.Signals.XData = [0 5 5 6 6 100]
      | sbobj.Groups.Signals.YData = [0 0 0.1 0.1 0 0]
      | sbobj.Groups.TimeRange = [0 100]
  Signal 1 : Outport  Tag=STV Outport
  wires:
  Demux/1 -> Signal 1/1
  FromWs/1 -> Demux/1

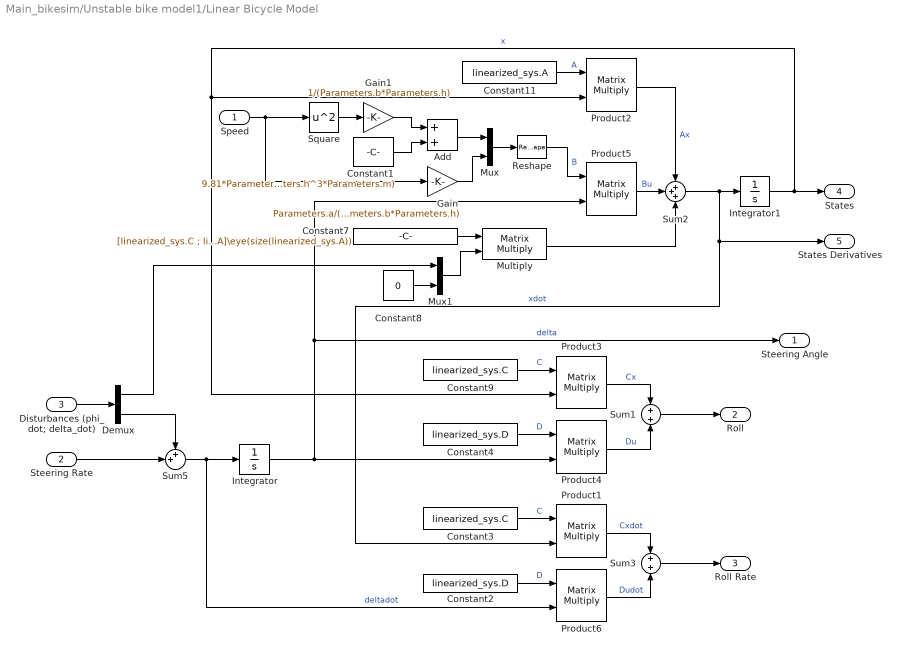
== system Main_bikesim/Unstable bike model1/Linear Bicycle Model ==
  Speed : Inport
  Steering Rate : Inport  Port=2
  Disturbances (phi_dot; delta_dot) : Inport  Port=3
  Add : Sum
  Constant1 : Constant  Value=9.81*Parameters.inertia_front/(Parameters.h^3*Parameters.m)
  Constant11 : Constant  Value=linearized_sys.A  VectorParams1D=off
  Constant2 : Constant  Value=linearized_sys.D  VectorParams1D=off
  Constant3 : Constant  Value=linearized_sys.C  VectorParams1D=off
  Constant4 : Constant  Value=linearized_sys.D  VectorParams1D=off
  Constant7 : Constant  Value=[linearized_sys.C ; linearized_sys.C*linearized_sys.A]\eye(size(linearized_sys.A))  VectorParams1D=off
  Constant8 : Constant  Value=0
  Constant9 : Constant  Value=linearized_sys.C  VectorParams1D=off
  Demux : Demux  Outputs=2
  Gain : Gain  Gain=Parameters.a/(Parameters.b*Parameters.h)
  Gain1 : Gain  Gain=1/(Parameters.b*Parameters.h)
  Integrator : Integrator  InitialCondition=Initial_State.steering
  Integrator1 : Integrator  InitialCondition=[linearized_sys.C ; linearized_sys.C*linearized_sys.A]\[Initial_State.roll ; Initial_State.roll_rate]
  Multiply : Product  Multiplication=Matrix(*)
  Mux : Mux  Inputs=2
  Mux1 : Mux  Inputs=2
  Product{1..6} (6 alike) : Product  SCDEnableBlockLinearizationSpecification=on  Multiplication=Matrix(*)
  Reshape : Reshape  OutputDimensionality=Customize  OutputDimensions=[size(linearized_sys.B,1),size(linearized_sys.B,2)]
  Square : Math  Operator=square  SignedPower=on
  Sum1 : Sum
  Sum2 : Sum  Inputs=+++
  Sum3 : Sum
  Sum5 : Sum  Inputs=++|
  Steering Angle : Outport  VectorParamsAs1DForOutWhenUnconnected=off
  Roll : Outport  Port=2  VectorParamsAs1DForOutWhenUnconnected=off
  Roll Rate : Outport  Port=3  VectorParamsAs1DForOutWhenUnconnected=off
  States : Outport  Port=4  VectorParamsAs1DForOutWhenUnconnected=off
  States Derivatives : Outport  Port=5  VectorParamsAs1DForOutWhenUnconnected=off
  wires:
  Product5/1 -> Sum2/2  "Bu"
  Constant11/1 -> Product2/1  "A"
  Sum2/1 -> Product1/2, States Derivatives/1, Integrator1/1  "xdot"
  Product2/1 -> Sum2/1  "Ax"
  Sum1/1 -> Roll/1
  Reshape/1 -> Product5/1  "B"
  Steering Rate/1 -> Sum5/2
  Product4/1 -> Sum1/2  "Du"
  Product3/1 -> Sum1/1  "Cx"
  Gain1/1 -> Add/1
  Constant1/1 -> Add/2
  Mux/1 -> Reshape/1
  Add/1 -> Mux/1
  Gain/1 -> Mux/2
  Speed/1 -> Square/1, Gain/1
  Square/1 -> Gain1/1
  Disturbances (phi_dot; delta_dot)/1 -> Demux/1
  Sum5/1 -> Integrator/1, Product6/2  "deltadot"
  Multiply/1 -> Sum2/3
  Demux/1 -> Mux1/1
  Constant7/1 -> Multiply/1
  Mux1/1 -> Multiply/2
  Constant8/1 -> Mux1/2
  Demux/2 -> Sum5/1
  Constant9/1 -> Product3/1  "C"
  Constant4/1 -> Product4/1  "D"
  Sum3/1 -> Roll Rate/1
  Integrator1/1 -> States/1, Product2/2, Product3/2  "x"
  Product6/1 -> Sum3/2  "Dudot"
  Constant3/1 -> Product1/1  "C"
  Product1/1 -> Sum3/1  "Cxdot"
  Constant2/1 -> Product6/1  "D"
  Integrator/1 -> Product5/2, Steering Angle/1, Product4/2  "delta"

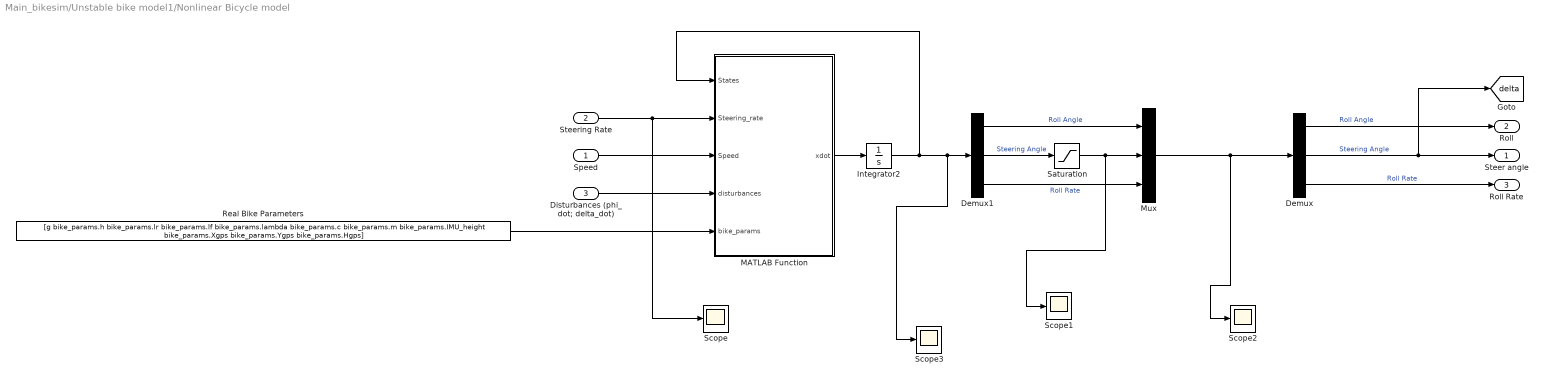
== system Main_bikesim/Unstable bike model1/Nonlinear Bicycle model ==
  Speed : Inport
  Steering Rate : Inport  Port=2
  Disturbances (phi_dot; delta_dot) : Inport  Port=3
  Demux : Demux  Outputs=3
  Demux1 : Demux  Outputs=3
  Integrator2 : Integrator  InitialCondition=[initial_state.roll ; initial_state.steering ; initial_state.roll_rate]
  MATLAB Function : MATLAB Function  TreatAsAtomicUnit=on
  Mux : Mux  Inputs=3
  Real Bike Parameters : Constant  Value=[g bike_params.h bike_params.lr bike_params.lf bike_params.lambda bike_params.c bike_params.m bike_params.IMU_height bike_params.Xgps bike_params.Ygps bike_params.Hgps]  SampleTime=Ts
  Saturation : Saturate  UpperLimit=deg2rad(48.7)  LowerLimit=-deg2rad(57.3)
  Scope{,1..3} (4 alike) : Scope
  Steer angle : Outport  VectorParamsAs1DForOutWhenUnconnected=off
  Roll : Outport  Port=2  VectorParamsAs1DForOutWhenUnconnected=off
  Roll Rate : Outport  Port=3  VectorParamsAs1DForOutWhenUnconnected=off
  tag scope: delta=global
  wires:
  Steering Rate/1 -> Scope/1, MATLAB Function/2(Steering_rate)
  Disturbances (phi_dot; delta_dot)/1 -> MATLAB Function/4(disturbances)
  Real Bike Parameters/1 -> MATLAB Function/5(bike_params)
  MATLAB Function/1(xdot) -> Integrator2/1
  Speed/1 -> MATLAB Function/3(Speed)
  Demux/1 -> Roll/1  "Roll Angle"
  Demux/3 -> Roll Rate/1  "Roll Rate"
  Demux/2 -> Steer angle/1, [delta]  "Steering Angle"
  Demux1/2 -> Saturation/1  "Steering Angle"
  Demux1/1 -> Mux/1  "Roll Angle"
  Demux1/3 -> Mux/3  "Roll Rate"
  Saturation/1 -> Scope1/1, Mux/2
  Integrator2/1 -> MATLAB Function/1(States), Scope3/1, Demux1/1
  Mux/1 -> Scope2/1, Demux/1

== system Main_bikesim/Unstable bike model1/Track bycicle pose ==
  Speed : Inport
  Steer angle : Inport  Port=2
  Constant : Constant  Value=[bike_params.lr bike_params.lf bike_params.lambda]
  Derivative of positions : MATLAB Function  TreatAsAtomicUnit=on
  Integrator with Wrapped State (between -pi & pi) : eeGeneralControl/Integrator with Wrapped State (Discrete or Continuous)  LabelModeActiveChoice=Discrete  WrappedStateUpperValue=pi  WrappedStateLowerValue=-pi  x0=initial_state_estimate.heading  Ts=Ts
  Integrator1 : Integrator  InitialCondition=initial_state_estimate.x
  Integrator2 : Integrator  InitialCondition=initial_state_estimate.y
  MATLAB Function : MATLAB Function  TreatAsAtomicUnit=on
  Mux : Mux  Inputs=3
  Pose : Outport
  wires:
  Derivative of positions/2(Ydot) -> Integrator2/1  "Ydot"
  Steer angle/1 -> MATLAB Function/2(steer_angle)
  Integrator2/1 -> Mux/2
  Mux/1 -> Pose/1
  Derivative of positions/1(Xdot) -> Integrator1/1  "Xdot"
  Speed/1 -> MATLAB Function/1(Speed), Derivative of positions/1(Speed)
  Integrator1/1 -> Mux/1
  MATLAB Function/1(beta) -> Derivative of positions/2(beta)
  Constant/1 -> MATLAB Function/3(bike_params)
  MATLAB Function/2(psi_dot) -> Integrator with Wrapped State (between -pi & pi)/1
  Integrator with Wrapped State (between -pi & pi)/1 -> Derivative of positions/3(psi), Mux/3

== matlab function Main_bikesim/Sensors1/Define true sensor positions on the bike ==
  data: bike_params input; pose input; pose_corrected output
function pose_corrected  = fcn(bike_params, pose)
pose_corrected = pose;

gpsX = bike_params(1); % measured offset of GPS parallel to bike
gpsY = bike_params(2); % measured offset of GPS perpendicular to bike
gpsH = bike_params(3); % measured offset of GPS from ground to GPS

% define pose_l
pose_l = pose;

% Transform to local frame
    pose_l(1) =  pose(1) * cos(pose(3)) + pose(2) * sin(pose(3));
    pose_l(2) = -pose(1) * sin(pose(3)) + pose(2) * cos(pose(3)); 

% define actual positions of GPS 
% pose1 = difference in x in local frame
% pose2 = difference in y in local frame
    pose_l(1) = pose_l(1) + gpsX;
    pose_l(2) = pose_l(2) + gpsY + gpsH*sin(pose(4));

% define actual positions of IMU 


% Transform back to global frame
    pose(1) = pose_l(1) * cos(pose(3)) - pose_l(2) * sin(pose(3));
    pose(2) = pose_l(1) * sin(pose(3)) + pose_l(2) * cos(pose(3));

pose_corrected(1) = pose(1);
pose_corrected(2) = pose(2);
